simulink library "Radiator"  (Simulink 8.2)
settings: Solver=ode45  StartTime=0.0  StopTime=10.0  RelTol=1e-3
libraries: carnot x2
settings Model: Creator=lena.frank  LastModifiedBy=drhf

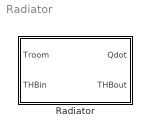
== system Radiator ==
  Radiator : Subsystem  mask(Radiator){pnom=500, dtnom=50, expo=1.3, mcap=5*4182, tini=20, lin=0, qua=1000}
      mask prompts: pnom "nominal power in W"; dtnom "nominal temperature difference in K"; expo "radiator exponent (> 0)"; mcap "mass * capacity per unit in J/K"; tini "initial temperature in degree Celsius"; lin "linear pressure drop dependace of massflow in Pa*s/kg"; qua "quadratic pressure drop dependace of massflow in Pa*s²/kg²"
      mask help:
      | Calculates the power of a radiator according to the nominal power the and the temperature difference (EN 442).
      | Qdot = Qdot_nom * (Tdiff/Tdiff_nom)^n
      | The thermal capacity of the radiator is modeled by a 1-node capacity.
      | mcp*dTnode/dt = mdot*cp*(Tin-Tnode)-Qdot
      | In difference to EN 442 the outlet temperature is Tnode. Tnode is not calculated as average temperature of inlet and outlet.
      | A quadratic pressure drop is applied to the fluid flow.
      mask Help: web(['file:///' fullfile(path_carnot('help'),'Radiator.html')],'-helpbrowser')
      mask Display:
      | plot(-20,0,120,90,[20 90 90 20 20],[20 20 70 70 20],[30 30],[25 65],[40 40],[25 65],[50 50],[25 65],[60 60],[25 65],[70 70],[25 65],[80 80],[25 65],[15 20],[25 25],[15 20],[65 65])
      | port_label('input',1,'Troom')
      | port_label('input',2,'THB')
      | port_label('output',1,'Qdot')
      | port_label('output',2,'THB')

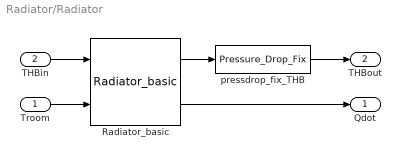
== system Radiator/Radiator ==
  Troom : Inport
  THBin : Inport  Port=2
  Radiator_basic : carnot/Basic/Thermal_Models/Radiator_basic  pnomEN=pnom  dtnomEN=dtnom  expo=expo  mcp=mcap
  pressdrop_fix_THB : carnot/Basic/Pressure_Drop/Pressure_Drop_Fix  con=0  lin=lin  qua=qua
  Qdot : Outport
  THBout : Outport  Port=2
  wires:
  Radiator_basic/2 -> Qdot/1
  Troom/1 -> Radiator_basic/2
  THBin/1 -> Radiator_basic/1
  Radiator_basic/1 -> pressdrop_fix_THB/1
  pressdrop_fix_THB/1 -> THBout/1
